simulink model "Part9"  (R2021a)
settings: Solver=VariableStepAuto  StartTime=0.0  StopTime=10.0  RelTol=1e-3
undefined symbols (not defined in the file): A, B, C, k, ka, L, x0
settings Model: Creator=ASUS  LastModifiedBy=ASUS

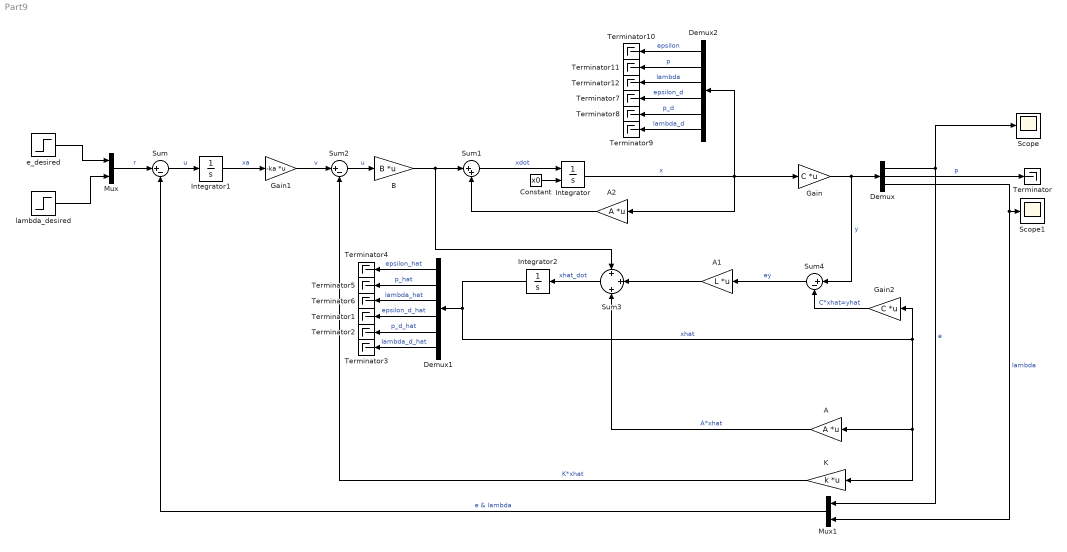
== system Part9 ==
  A : Gain  Gain=A  Multiplication=Matrix(K*u)
  A1 : Gain  Gain=L  Multiplication=Matrix(K*u)
  A2 : Gain  Gain=A  Multiplication=Matrix(K*u)
  B : Gain  Gain=B  Multiplication=Matrix(K*u)
  Constant : Constant  Value=x0
  Demux : Demux  Outputs=3
  Demux1 : Demux  Outputs=6
  Demux2 : Demux  Outputs=6
  Gain : Gain  Gain=C  Multiplication=Matrix(K*u)
  Gain1 : Gain  Gain=-ka  Multiplication=Matrix(K*u)
  Gain2 : Gain  Gain=C  Multiplication=Matrix(K*u)
  Integrator : Integrator  InitialConditionSource=external
  Integrator1 : Integrator
  Integrator2 : Integrator
  K : Gain  Gain=k  Multiplication=Matrix(K*u)
  Mux : Mux  Inputs=2
  Mux1 : Mux  Inputs=2
  Scope : Scope
  Scope1 : Scope
  Sum : Sum  Inputs=|+-
  Sum1 : Sum  Inputs=|++
  Sum2 : Sum  Inputs=|+-
  Sum3 : Sum  Inputs=+|+|+
  Sum4 : Sum  Inputs=|+-
  Terminator{,1..12} (13 alike) : Terminator
  e_desired : Step  Time=0  After=0.03  SampleTime=0
  lambda_desired : Step  Time=0  After=0.05  SampleTime=0
  wires:
  Sum2/1 -> B/1  "u"
  Demux/2 -> Terminator/1  "p"
  Mux1/1 -> Sum/2  "e & lambda"
  Gain1/1 -> Sum2/1  "v"
  Sum/1 -> Integrator1/1  "u"
  Demux/3 -> Mux1/2, Scope1/1  "lambda"
  Integrator/1 -> Demux2/1, Gain/1, A2/1  "x"
  Gain/1 -> Demux/1, Sum4/1  "y"
  Integrator1/1 -> Gain1/1  "xa"
  A/1 -> Sum3/3  "A*xhat"
  Sum1/1 -> Integrator/1  "xdot"
  K/1 -> Sum2/2  "K*xhat"
  Demux/1 -> Scope/1, Mux1/1  "e"
  B/1 -> Sum3/1, Sum1/1
  Mux/1 -> Sum/1  "r"
  A1/1 -> Sum3/2
  Sum3/1 -> Integrator2/1  "xhat_dot"
  Integrator2/1 -> Demux1/1, Gain2/1, K/1, A/1  "xhat"
  Gain2/1 -> Sum4/2  "C*xhat=yhat"
  Sum4/1 -> A1/1  "ey"
  A2/1 -> Sum1/2
  e_desired/1 -> Mux/1
  lambda_desired/1 -> Mux/2
  Demux1/4 -> Terminator1/1  "epsilon_d_hat"
  Demux1/5 -> Terminator2/1  "p_d_hat"
  Demux1/6 -> Terminator3/1  "lambda_d_hat"
  Demux1/3 -> Terminator6/1  "lambda_hat"
  Demux1/2 -> Terminator5/1  "p_hat"
  Demux1/1 -> Terminator4/1  "epsilon_hat"
  Demux2/1 -> Terminator10/1  "epsilon"
  Demux2/2 -> Terminator11/1  "p"
  Demux2/3 -> Terminator12/1  "lambda"
  Demux2/6 -> Terminator9/1  "lambda_d"
  Demux2/5 -> Terminator8/1  "p_d"
  Demux2/4 -> Terminator7/1  "epsilon_d"
  Constant/1 -> Integrator/2
